simulink model "main_RI_LIEKF_GNSSOutrage"  (R2023a)
settings: Solver=FixedStepAuto  StartTime=0.0  StopTime=220  FixedStep=0.01  RelTol=1e-3
InitFcn:
  | initNavigation0612_AOA;
values from neighbouring files (symbols this model uses):
  CF_enable = 0    [initNavigation.m]
  dt = 0.01    [initNavigation.m]
  dtDelay = -0.03    [initNavigation.m]
  g0 = 9.795    [initNavigation.m]
  gam0_rad = 0/57.3    (= 0)    [initNavigation.m]
  GNSSoutragetime = 90    [initNavigation.m]
  H_sensor_type = 0    [initNavigation.m]
  KF_enable = 1    [initNavigation.m]
  P0 = diag([1*ones(3,1);0.01*ones(3,1);0.1*ones(3,1);0.001*ones(3,1);0.00001*ones(3,1)])    [initNavigation.m]
  P0_RIEKF = diag([1*ones(3,1);0.01*ones(3,1);0.1*ones(3,1);0.001*ones(3,1);0.00001*ones(3,1);      0.01*ones(3,1);[0;2;2]/57.3;[0.1;0.1;0.1]])^2    [initNavigation.m]
  pd0 = 0    [initNavigation.m]
  pe0 = 0    [initNavigation.m]
  phi0_rad = 0/57.3    (= 0)    [initNavigation.m]
  pn0 = 0    [initNavigation.m]
  psi = -178    [initNavigation.m]
  psi0_rad = 0/57.3    (= 0)    [initNavigation.m]
  state_dim = 24    [initNavigation.m]
  Time = 0:0.01:(size(traindata.AttackAngle,1) - 1)*0.01    [NNLiftCoefficientFit.m]
  vd0 = 0    [initNavigation.m]
  ve0 = 0    [initNavigation.m]
  vn0 = 0    [initNavigation.m]
undefined symbols (not defined in the file or in its folder): DiscIntNeverNeededParam, Discrete, INS_CONST, INS_EXPORT, INS_PARAM, magnitude, p, param, pInitialization, sys
libraries: simulink_extras x94, simulink x82, dspstat3 x70, sharedtransform x60, ctrlSharedLib x36, sharedTrackingLibrary x22, matrix_library x15, FMT_Model_Lib x13, deeplib x8, dspsolvers x4, vrlib x4, aerolibconvert2 x1
(part 11 of 28)

== system main_RI_LIEKF_GNSSOutrage/State estimation/LI EKF2/Error State Kalman Filter/Extended Kalman Filter1 ==
  Q : Inport
  Enable1 : Inport  Port=2
  y1 : Inport  Port=3
  R1 : Inport  Port=4
  Enable2 : Inport  Port=5
  y2 : Inport  Port=6
  R2 : Inport  Port=7
  Enable3 : Inport  Port=8
  y3 : Inport  Port=9
  R3 : Inport  Port=10
  Enable4 : Inport  Port=11
  y4 : Inport  Port=12
  R4 : Inport  Port=13
  BlockOrdering : Constant  Value=true()  OutDataTypeStr=boolean
  Correct1 : Subsystem  AncestorBlock=sharedTrackingLibrary/Extras/EKFCorrect  TreatAsAtomicUnit=on  SystemSampleTime=p.SampleTimes.MeasurementFcn(1)  mask(EKFCorrect){ProcessedMaskData=p}
      mask init: same as main_RI_LIEKF_GNSSOutrage/State estimation/0609bk/Error State Kalman Filter/Extended Kalman Filter1/Correct1
      settings: LibrarySourceBlock=sharedTrackingLibrary/Extras/EKFCorrect
  Correct2 : sharedTrackingLibrary/Extras/EKFCorrect  ProcessedMaskData=p
  Correct3 : sharedTrackingLibrary/Extras/EKFCorrect  ProcessedMaskData=p
  Correct4 : sharedTrackingLibrary/Extras/EKFCorrect  ProcessedMaskData=p
  DataStoreMemory - P : DataStoreMemory  DataStoreName=P  InitialValue=p.InitialCovariance  ShowAdditionalParam=off  OutDataTypeStr=p.DataType
  DataStoreMemory - x : DataStoreMemory  DataStoreName=x  InitialValue=p.InitialState  ShowAdditionalParam=off  OutDataTypeStr=p.DataType
  DataTypeConversion_Enable{1..4} (4 alike) : DataTypeConversion  OutDataTypeStr=boolean  SaturateOnIntegerOverflow=off  RndMeth=Floor
  DataTypeConversion_Q : DataTypeConversion  OutDataTypeStr=p.DataType  SaturateOnIntegerOverflow=off  RndMeth=Floor
  DataTypeConversion_R{1..4} (4 alike) : DataTypeConversion  OutDataTypeStr=p.DataType  SaturateOnIntegerOverflow=off  RndMeth=Floor
  DataTypeConversion_uMeas{1..4} (4 alike) : DataTypeConversion  OutDataTypeStr=p.DataType  SaturateOnIntegerOverflow=off  RndMeth=Floor
  DataTypeConversion_uState : DataTypeConversion  OutDataTypeStr=p.DataType  SaturateOnIntegerOverflow=off  RndMeth=Floor
  DataTypeConversion_y{1..4} (4 alike) : DataTypeConversion  OutDataTypeStr=p.DataType  SaturateOnIntegerOverflow=off  RndMeth=Floor
  MeasurementFcn1Inputs : Constant  Value=0  OutDataTypeStr=p.DataType  SampleTime=p.SampleTimes.MeasurementFcn(1)
  MeasurementFcn2Inputs : Constant  OutDataTypeStr=p.DataType  SampleTime=p.SampleTimes.MeasurementFcn(2)
  MeasurementFcn3Inputs : Constant  OutDataTypeStr=p.DataType  SampleTime=p.SampleTimes.MeasurementFcn(3)
  MeasurementFcn4Inputs : Constant  OutDataTypeStr=p.DataType  SampleTime=p.SampleTimes.MeasurementFcn(4)
  Output : Subsystem  TreatAsAtomicUnit=on  SystemSampleTime=p.SampleTimes.Output
  Predict : Subsystem  TreatAsAtomicUnit=on  SystemSampleTime=p.SampleTimes.StateTransitionFcn  mask(EKFPredict){ProcessedMaskData=p}
      mask init: same as main_RI_LIEKF_GNSSOutrage/State estimation/0609bk/Error State Kalman Filter/Extended Kalman Filter1/Predict
  StateTransitionFcnInputs : Constant  Value=0  OutDataTypeStr=p.DataType  SampleTime=p.SampleTimes.StateTransitionFcn
  checkMeasurementFcn1Signals : S-Function  FunctionName=ekfukfCheckSignals  Parameters=signalCheck.BlockPath, signalCheck.MeasurementFcn{1}.PortNames, signalCheck.MeasurementFcn{1}.SampleTime, signalCheck.DataType, signalCheck.MeasurementFcn{1}.PortDimensions, 1, signalCheck.MeasurementFcn{1}.HasAdditiveNoise  SFunctionDeploymentMode=off  EnableBusSupport=off
  checkMeasurementFcn2Signals : S-Function  FunctionName=ekfukfCheckSignals  Parameters=signalCheck.BlockPath, signalCheck.MeasurementFcn{2}.PortNames, signalCheck.MeasurementFcn{2}.SampleTime, signalCheck.DataType, signalCheck.MeasurementFcn{2}.PortDimensions, 1, signalCheck.MeasurementFcn{2}.HasAdditiveNoise  SFunctionDeploymentMode=off  EnableBusSupport=off
  checkMeasurementFcn3Signals : S-Function  FunctionName=ekfukfCheckSignals  Parameters=signalCheck.BlockPath, signalCheck.MeasurementFcn{3}.PortNames, signalCheck.MeasurementFcn{3}.SampleTime, signalCheck.DataType, signalCheck.MeasurementFcn{3}.PortDimensions, 1, signalCheck.MeasurementFcn{3}.HasAdditiveNoise  SFunctionDeploymentMode=off  EnableBusSupport=off
  checkMeasurementFcn4Signals : S-Function  FunctionName=ekfukfCheckSignals  Parameters=signalCheck.BlockPath, signalCheck.MeasurementFcn{4}.PortNames, signalCheck.MeasurementFcn{4}.SampleTime, signalCheck.DataType, signalCheck.MeasurementFcn{4}.PortDimensions, 1, signalCheck.MeasurementFcn{4}.HasAdditiveNoise  SFunctionDeploymentMode=off  EnableBusSupport=off
  checkStateTransitionFcnSignals : S-Function  FunctionName=ekfukfCheckSignals  Parameters=signalCheck.BlockPath, signalCheck.StateTransitionFcn.PortNames, signalCheck.StateTransitionFcn.SampleTime, signalCheck.DataType, signalCheck.StateTransitionFcn.PortDimensions, 0, signalCheck.StateTransitionFcn.HasAdditiveNoise  SFunctionDeploymentMode=off  EnableBusSupport=off
  xhat : Outport  VectorParamsAs1DForOutWhenUnconnected=off
  P : Outport  Port=2
  wires:
  Correct4/1 -> [AfterCorrect]
  Correct3/1 -> Correct4/4
  MeasurementFcn4Inputs/1 -> checkMeasurementFcn4Signals/4, DataTypeConversion_uMeas4/1
  R4/1 -> checkMeasurementFcn4Signals/3, DataTypeConversion_R4/1
  y4/1 -> checkMeasurementFcn4Signals/2, DataTypeConversion_y4/1
  Enable4/1 -> checkMeasurementFcn4Signals/1, DataTypeConversion_Enable4/1
  DataTypeConversion_uMeas4/1 -> Correct4/3
  DataTypeConversion_R4/1 -> Correct4/2
  DataTypeConversion_y4/1 -> Correct4/1
  DataTypeConversion_Enable4/1 -> Correct4/Enable
  Correct2/1 -> Correct3/4
  MeasurementFcn3Inputs/1 -> checkMeasurementFcn3Signals/4, DataTypeConversion_uMeas3/1
  R3/1 -> checkMeasurementFcn3Signals/3, DataTypeConversion_R3/1
  y3/1 -> checkMeasurementFcn3Signals/2, DataTypeConversion_y3/1
  Enable3/1 -> checkMeasurementFcn3Signals/1, DataTypeConversion_Enable3/1
  DataTypeConversion_uMeas3/1 -> Correct3/3
  DataTypeConversion_R3/1 -> Correct3/2
  DataTypeConversion_y3/1 -> Correct3/1
  DataTypeConversion_Enable3/1 -> Correct3/Enable
  Correct1/1(yBlockOrdering) -> Correct2/4
  MeasurementFcn2Inputs/1 -> checkMeasurementFcn2Signals/4, DataTypeConversion_uMeas2/1
  R2/1 -> checkMeasurementFcn2Signals/3, DataTypeConversion_R2/1
  y2/1 -> checkMeasurementFcn2Signals/2, DataTypeConversion_y2/1
  Enable2/1 -> checkMeasurementFcn2Signals/1, DataTypeConversion_Enable2/1
  DataTypeConversion_uMeas2/1 -> Correct2/3
  DataTypeConversion_R2/1 -> Correct2/2
  DataTypeConversion_y2/1 -> Correct2/1
  DataTypeConversion_Enable2/1 -> Correct2/Enable
  [AfterOutput] -> Predict/3(uBlockOrdering)
  Output/3(yBlockOrdering) -> [AfterOutput]
  [AfterCorrect] -> Output/1(uBlockOrdering)
  [FirstOperation] -> Correct1/4(uBlockOrdering)
  BlockOrdering/1 -> [FirstOperation]
  DataTypeConversion_uMeas1/1 -> Correct1/3(uMeas)
  DataTypeConversion_R1/1 -> Correct1/2(R)
  MeasurementFcn1Inputs/1 -> DataTypeConversion_uMeas1/1, checkMeasurementFcn1Signals/4
  DataTypeConversion_y1/1 -> Correct1/1(yMeas)
  DataTypeConversion_uState/1 -> Predict/2(uState)
  StateTransitionFcnInputs/1 -> DataTypeConversion_uState/1, checkStateTransitionFcnSignals/2
  Output/2(P) -> P/1
  DataTypeConversion_Enable1/1 -> Correct1/Enable
  Enable1/1 -> DataTypeConversion_Enable1/1, checkMeasurementFcn1Signals/1
  DataTypeConversion_Q/1 -> Predict/1(Q)
  Q/1 -> DataTypeConversion_Q/1, checkStateTransitionFcnSignals/1
  R1/1 -> DataTypeConversion_R1/1, checkMeasurementFcn1Signals/3
  y1/1 -> DataTypeConversion_y1/1, checkMeasurementFcn1Signals/2
  Output/1(x) -> xhat/1

== system main_RI_LIEKF_GNSSOutrage/State estimation/LI EKF2/Error State Kalman Filter/Simulink Function - GPS Measurements ==
  Rbn : Inport
  vn : Inport  Port=2
  pn : Inport  Port=3
  GPSMeasurementFcn_LIEKF : TriggerPort  TriggerType=function-call  IsSimulinkFunction=on  FunctionName=GPSMeasurementFcn_LIEKF  VariantControl=Variant
  Add : Sum
  Data Type Conversion1 : DataTypeConversion  OutDataTypeStr=single  SaturateOnIntegerOverflow=off  RndMeth=Floor
  MATLAB Function : MATLAB Function  TreatAsAtomicUnit=on
  MATLAB Function1 : MATLAB Function  Commented=on  TreatAsAtomicUnit=on
  Product : Product  Multiplication=Matrix(*)
  pn1 : InportShadow  Port=3
  vn1 : InportShadow  Port=2
  x : ArgIn  DisableCoverage=on  OutDataTypeStr=single  PortDimensions=state_dim  ArgumentName=x
  v : ArgIn  DisableCoverage=on  Port=2  OutDataTypeStr=single  PortDimensions=6  ArgumentName=v
  y : ArgOut  DisableCoverage=on  OutDataTypeStr=single  PortDimensions=6  ArgumentName=y
  wires:
  MATLAB Function/1(H) -> Data Type Conversion1/1
  Product/1 -> Add/1
  Add/1 -> y/1
  vn/1 -> MATLAB Function/1(vn)
  Rbn/1 -> MATLAB Function1/1(Rbn)
  vn1/1 -> MATLAB Function1/2(vn)
  pn1/1 -> MATLAB Function1/3(pn)
  x/1 -> Product/2
  v/1 -> Add/2
  pn/1 -> MATLAB Function/2(pn)
  Data Type Conversion1/1 -> Product/1

== system main_RI_LIEKF_GNSSOutrage/State estimation/LI EKF2/Error State Kalman Filter/Simulink Function - GPS Measurements1 ==
  vn : Inport
  pn : Inport  Port=2
  BaroMeasurementFcn_LIEKF : TriggerPort  TriggerType=function-call  IsSimulinkFunction=on  FunctionName=BaroMeasurementFcn_LIEKF  VariantControl=Variant
  Add : Sum
  Data Type Conversion1 : DataTypeConversion  OutDataTypeStr=single  SaturateOnIntegerOverflow=off  RndMeth=Floor
  MATLAB Function : MATLAB Function  TreatAsAtomicUnit=on
  Product : Product  Multiplication=Matrix(*)
  x : ArgIn  DisableCoverage=on  OutDataTypeStr=single  PortDimensions=state_dim  ArgumentName=x
  v : ArgIn  DisableCoverage=on  Port=2  OutDataTypeStr=single  ArgumentName=v
  y : ArgOut  DisableCoverage=on  OutDataTypeStr=single  ArgumentName=y
  wires:
  MATLAB Function/1(H_baro) -> Data Type Conversion1/1
  Product/1 -> Add/1
  Add/1 -> y/1
  vn/1 -> MATLAB Function/1(vn)
  x/1 -> Product/2
  v/1 -> Add/2
  pn/1 -> MATLAB Function/2(pn)
  Data Type Conversion1/1 -> Product/1

== system main_RI_LIEKF_GNSSOutrage/State estimation/LI EKF2/Error State Kalman Filter/Simulink Function - GPS Measurements2 ==
  Rbn : Inport
  Magn : Inport  Port=2
  xstate : Inport  Port=3
  MagnMeasurementFcn_LIEKF : TriggerPort  TriggerType=function-call  IsSimulinkFunction=on  FunctionName=MagnMeasurementFcn_LIEKF  VariantControl=Variant
  Add : Sum
  Data Type Conversion1 : DataTypeConversion  OutDataTypeStr=single  SaturateOnIntegerOverflow=off  RndMeth=Floor
  MATLAB Function : MATLAB Function  TreatAsAtomicUnit=on
  Product : Product  Multiplication=Matrix(*)
  Selector : Selector  InputPortWidth=state_dim  IndexOptions=Index vector (dialog)  Indices=[1 2 3]  OutputSizes=1
  x : ArgIn  DisableCoverage=on  OutDataTypeStr=single  PortDimensions=state_dim  ArgumentName=x
  v : ArgIn  DisableCoverage=on  Port=2  OutDataTypeStr=single  PortDimensions=3  ArgumentName=v
  y : ArgOut  DisableCoverage=on  OutDataTypeStr=single  PortDimensions=3  ArgumentName=y
  wires:
  MATLAB Function/1(H) -> Data Type Conversion1/1
  Product/1 -> Add/1
  Add/1 -> y/1
  Magn/1 -> MATLAB Function/2(Magn)
  x/1 -> Product/2
  v/1 -> Add/2
  Data Type Conversion1/1 -> Product/1
  Rbn/1 -> MATLAB Function/1(Rbn)
  xstate/1 -> Selector/1
  Selector/1 -> MATLAB Function/3(dtheta)

== system main_RI_LIEKF_GNSSOutrage/State estimation/LI EKF2/Error State Kalman Filter/Simulink Function - GPS Measurements3 ==
  Rbn : Inport
  vn : Inport  Port=2
  Rab : Inport  Port=3
  vel_wind_NED : Inport  Port=4
  AirspeedMeasurementFcn_LIEKF : TriggerPort  TriggerType=function-call  IsSimulinkFunction=on  FunctionName=AirspeedMeasurementFcn_LIEKF  VariantControl=Variant
  Add : Sum
  Data Type Conversion1 : DataTypeConversion  OutDataTypeStr=single  SaturateOnIntegerOverflow=off  RndMeth=Floor
  MATLAB Function : MATLAB Function  TreatAsAtomicUnit=on
  Product : Product  Multiplication=Matrix(*)
  x : ArgIn  DisableCoverage=on  OutDataTypeStr=single  PortDimensions=state_dim  ArgumentName=x
  v : ArgIn  DisableCoverage=on  Port=2  OutDataTypeStr=single  PortDimensions=3  ArgumentName=v
  y : ArgOut  DisableCoverage=on  OutDataTypeStr=single  PortDimensions=3  ArgumentName=y
  wires:
  MATLAB Function/1(H) -> Data Type Conversion1/1
  Product/1 -> Add/1
  Add/1 -> y/1
  x/1 -> Product/2
  v/1 -> Add/2
  Data Type Conversion1/1 -> Product/1
  Rbn/1 -> MATLAB Function/1(Rbn)
  vn/1 -> MATLAB Function/3(vn)
  Rab/1 -> MATLAB Function/2(Rab)
  vel_wind_NED/1 -> MATLAB Function/4(v_wind)

== system main_RI_LIEKF_GNSSOutrage/State estimation/LI EKF2/Error State Kalman Filter/Simulink Function - State Transition ==
  DCM_b_n : Inport
  wxyz : Inport  Port=2  PortDimensions=[3,1]
  axyz : Inport  Port=3  PortDimensions=[3,1]
  stateTransitionFcn_LIEKF : TriggerPort  TriggerType=function-call  IsSimulinkFunction=on  FunctionName=stateTransitionFcn_LIEKF  VariantControl=Variant
  Add : Sum
  Cal Phi : Subsystem
  Constant : Constant  Value=dt  OutDataTypeStr=single
  Data Type Conversion1 : DataTypeConversion  OutDataTypeStr=single  SaturateOnIntegerOverflow=off  RndMeth=Floor
  Data Type Conversion6 : DataTypeConversion  OutDataTypeStr=single  SaturateOnIntegerOverflow=off  RndMeth=Floor
  MATLAB Function1 : MATLAB Function  TreatAsAtomicUnit=on
  Product1 : Product  Multiplication=Matrix(*)
  Product2 : Product  Multiplication=Matrix(*)
  x : ArgIn  DisableCoverage=on  OutDataTypeStr=single  PortDimensions=state_dim  ArgumentName=x
  w : ArgIn  Port=2  OutDataTypeStr=single  PortDimensions=cov_dim  ArgumentName=w
  xNext : ArgOut  DisableCoverage=on  OutDataTypeStr=single  PortDimensions=state_dim  ArgumentName=xNext
  wires:
  x/1 -> Product2/2
  Product2/1 -> Data Type Conversion6/1
  MATLAB Function1/1(G) -> Product1/1
  w/1 -> Product1/2
  Product1/1 -> Data Type Conversion1/1
  Add/1 -> xNext/1
  [DCM_b_n] -> MATLAB Function1/1(Rbn)
  Constant/1 -> MATLAB Function1/2(dt)
  DCM_b_n/1 -> [DCM_b_n]
  Cal Phi/1(Phi) -> Product2/1
  Data Type Conversion6/1 -> Add/2
  [DCM_b_n] -> Cal Phi/1(Rbn)
  wxyz/1 -> Cal Phi/2(wxyz)
  axyz/1 -> Cal Phi/3(axyz)
  Data Type Conversion1/1 -> Add/1

== system main_RI_LIEKF_GNSSOutrage/State estimation/LI EKF2/Error State Kalman Filter/Simulink Function - State Transition1 ==
  DCM_b_n : Inport
  wxyz : Inport  Port=2  PortDimensions=[3,1]
  axyz : Inport  Port=3  PortDimensions=[3,1]
  stateFcn_LIEKFJacobian : TriggerPort  TriggerType=function-call  IsSimulinkFunction=on  FunctionName=stateFcn_LIEKFJacobian  VariantControl=Variant
  Cal Phi : Subsystem
  Constant : Constant  Value=dt  OutDataTypeStr=single
  Data Type Conversion1 : DataTypeConversion  OutDataTypeStr=single  SaturateOnIntegerOverflow=off  RndMeth=Floor
  Data Type Conversion6 : DataTypeConversion  OutDataTypeStr=single  SaturateOnIntegerOverflow=off  RndMeth=Floor
  MATLAB Function1 : MATLAB Function  TreatAsAtomicUnit=on
  Terminator : Terminator
  Terminator1 : Terminator
  x : ArgIn  DisableCoverage=on  OutDataTypeStr=single  PortDimensions=state_dim  ArgumentName=x
  w : ArgIn  Port=2  OutDataTypeStr=single  PortDimensions=cov_dim  ArgumentName=w
  A : ArgOut  DisableCoverage=on  OutDataTypeStr=single  PortDimensions=[state_dim,state_dim]  ArgumentName=A
  G : ArgOut  Port=2  OutDataTypeStr=single  PortDimensions=[24,21]  ArgumentName=G
  wires:
  axyz/1 -> Cal Phi/3(a)
  wxyz/1 -> Cal Phi/2(w)
  [DCM_b_n] -> Cal Phi/1(Rbn)
  DCM_b_n/1 -> [DCM_b_n]
  Constant/1 -> MATLAB Function1/2(dt)
  [DCM_b_n] -> MATLAB Function1/1(Rbn)
  w/1 -> Terminator/1
  x/1 -> Terminator1/1
  MATLAB Function1/1(G) -> Data Type Conversion6/1
  Cal Phi/1(Phi) -> Data Type Conversion1/1
  Data Type Conversion6/1 -> G/1
  Data Type Conversion1/1 -> A/1

== system main_RI_LIEKF_GNSSOutrage/State estimation/LI EKF2/Error State Kalman Filter/Subsystem ==
  data : Inport
  Detect Change : simulink/Logic and Bit Operations/Detect Change  vinit=0  InputProcessing=Columns as channels (frame based)  OutDataTypeStr=boolean
  Selector : Selector  InputPortWidth=3  IndexOptions=Index vector (dialog)  Indices=[3]  OutputSizes=1
  Zero-Order Hold : ZeroOrderHold  SampleTime=0.2
  Zero-Order Hold1 : ZeroOrderHold  SampleTime=0.01
  flag : Outport
  wires:
  Zero-Order Hold1/1 -> Detect Change/1
  Detect Change/1 -> flag/1
  Selector/1 -> Zero-Order Hold1/1
  data/1 -> Zero-Order Hold/1
  Zero-Order Hold/1 -> Selector/1

== system main_RI_LIEKF_GNSSOutrage/State estimation/LI EKF2/Error State Kalman Filter/Subsystem1 ==
  Cbn : Inport
  v_I : Inport  Port=2
  v_G : Inport  Port=3
  p_I : Inport  Port=4
  p_G : Inport  Port=5
  Add1 : Sum  Inputs=+-
  Add2 : Sum  Inputs=+-
  Data Type Conversion : DataTypeConversion  OutDataTypeStr=single  SaturateOnIntegerOverflow=off  RndMeth=Floor
  Data Type Conversion2 : DataTypeConversion  OutDataTypeStr=single  SaturateOnIntegerOverflow=off  RndMeth=Floor
  Gain1 : Gain  Gain=-1
  Mux2 : Mux  Inputs=2
  Product : Product  Multiplication=Matrix(*)
  Product1 : Product  Multiplication=Matrix(*)
  Transpose : Math  Operator=transpose
  dv/dp : Outport
  wires:
  Gain1/1 -> dv/dp/1
  Mux2/1 -> Gain1/1
  Product1/1 -> Data Type Conversion/1
  Product/1 -> Data Type Conversion2/1
  Transpose/1 -> Product1/1, Product/1
  Cbn/1 -> Transpose/1
  Data Type Conversion2/1 -> Mux2/1
  v_G/1 -> Add2/2
  Data Type Conversion/1 -> Mux2/2
  p_I/1 -> Add1/1
  Add1/1 -> Product1/2
  Add2/1 -> Product/2
  v_I/1 -> Add2/1
  p_G/1 -> Add1/2

== system main_RI_LIEKF_GNSSOutrage/State estimation/LI EKF2/Error State Kalman Filter/Subsystem2 ==
  p_INS : Inport
  H_baro : Inport  Port=2
  Add : Sum
  dpZ : Outport
  wires:
  p_INS/1 -> Add/1
  H_baro/1 -> Add/2
  Add/1 -> dpZ/1

== system main_RI_LIEKF_GNSSOutrage/State estimation/LI EKF2/Error State Kalman Filter/Subsystem3 ==
  data : Inport
  Detect Change : simulink/Logic and Bit Operations/Detect Change  vinit=0  InputProcessing=Columns as channels (frame based)  OutDataTypeStr=boolean
  From Workspace1 : FromWorkspace  Commented=on  VariableName=[All.t',All.vn]
  From Workspace7 : FromWorkspace  VariableName=[All.t',All.lat]
  Selector : Selector  InputPortWidth=3  IndexOptions=Index vector (dialog)  Indices=[3]  OutputSizes=1
  flag : Outport
  wires:
  Detect Change/1 -> flag/1
  data/1 -> Selector/1
  From Workspace7/1 -> Detect Change/1  "lat"

== system main_RI_LIEKF_GNSSOutrage/State estimation/LI EKF2/Error State Kalman Filter/bak ==
  From1 : From  Commented=on  GotoTag=wxyz
  From11 : From  Commented=on  GotoTag=p_INS
  From14 : From  Commented=on  GotoTag=DCM_b_n
  From2 : From  Commented=on  GotoTag=fbxyz
  From3 : From  Commented=on  GotoTag=ZUPTenable
  From4 : From  Commented=on  GotoTag=v_INS
  From5 : From  Commented=on  GotoTag=fex
  From6 : From  Commented=on  GotoTag=DCM_b_n
  From9 : From  Commented=on  GotoTag=DCM_b_n
  Goto6 : Goto  Commented=on  GotoTag=ZUPTenable
  MATLAB Function1 : MATLAB Function  Commented=on  TreatAsAtomicUnit=on
  Memory1 : Memory  Commented=on
  RIEKF : MATLAB Function  Commented=on  TreatAsAtomicUnit=on
  Rate Transition2 : RateTransition  Commented=on  OutPortSampleTime=dt
  Scope10 : Scope  Commented=on  NumInputPorts=2
  Simulink Function - GPS Measurements1 : Subsystem  Commented=on  TreatAsAtomicUnit=on
  Simulink Function - GPS Measurements2 : Subsystem  Commented=on  TreatAsAtomicUnit=on
  Simulink Function - State Transition Jacobian : Subsystem  Commented=on  TreatAsAtomicUnit=on
  Unscented Kalman Filter1 : sharedTrackingLibrary/Unscented Kalman Filter  Commented=on  StateTransitionFcn=stateTransitionFcn_Dyn  HasAdditiveProcessNoise=Nonadditive  ProcessNoise=1  HasTimeVaryingProcessNoise=on  HasStateTransitionFcnExtraArgument=0  InitialState=zeros(18,1)  InitialStateCovariance=diag([1*ones(3,1);0.1*ones(3,1);0.001*ones(3,1);0.001*ones(6,1);0.1*ones(3,1)]);  Alpha=1e-2  Beta=2  Kappa=0  MeasurementFcn1=GPSMeasurementFcn_Dyn  HasMeasurementEnablePort1=on  HasAdditiveMeasurementNoise1=Nonadditive  MeasurementNoise1=1  HasTimeVaryingMeasurementNoise1=on  HasMeasurementFcnExtraArgument1=0  HasMeasurementWrapping1=off  MeasurementFcn2=DynamicMeasurementFcn_Dyn  HasMeasurementEnablePort2=on  HasAdditiveMeasurementNoise2=Nonadditive  MeasurementNoise2=1  HasTimeVaryingMeasurementNoise2=on  HasMeasurementFcnExtraArgument2=0  HasMeasurementWrapping2=off  MeasurementFcn3=myMeasurementFcn  HasMeasurementEnablePort3=off  HasAdditiveMeasurementNoise3=Additive  MeasurementNoise3=1  HasTimeVaryingMeasurementNoise3=off  HasMeasurementFcnExtraArgument3=0  HasMeasurementWrapping3=off  MeasurementFcn4=myMeasurementFcn  HasMeasurementEnablePort4=off  HasAdditiveMeasurementNoise4=Additive  MeasurementNoise4=1  HasTimeVaryingMeasurementNoise4=off  HasMeasurementFcnExtraArgument4=0  HasMeasurementWrapping4=off  MeasurementFcn5=myMeasurementFcn  HasMeasurementEnablePort5=off  HasAdditiveMeasurementNoise5=Additive  MeasurementNoise5=1  HasTimeVaryingMeasurementNoise5=off  HasMeasurementFcnExtraArgument5=0  HasMeasurementWrapping5=off  EnableMultirate=off  StateTransitionFcnSampleTime=1  MeasurementFcn1SampleTime=1  MeasurementFcn2SampleTime=1  MeasurementFcn3SampleTime=1  MeasurementFcn4SampleTime=1  MeasurementFcn5SampleTime=1  UseCurrentEstimator=on  OutputStateCovariance=on  DataType=single  SampleTime=0.01  NumberOfMeasurements=2
  Out1 : Outport
  wires:
  Memory1/1 -> MATLAB Function1/4(fex)
  Rate Transition2/1 -> Out1/1
  From1/1 -> MATLAB Function1/2(wxyz)
  MATLAB Function1/1(ZeroVelDetectFlag) -> Scope10/1, Goto6/1
  From5/1 -> Memory1/1
  From2/1 -> MATLAB Function1/3(fbxyz)
  From6/1 -> MATLAB Function1/1(Cbn)
  MATLAB Function1/2(ZeroVelDetectFlagold) -> Scope10/2
  From3/1 -> Rate Transition2/1
  From11/1 -> Simulink Function - State Transition Jacobian/3(pn)
  From9/1 -> Simulink Function - State Transition Jacobian/1(DCM_b_n)
  From4/1 -> Simulink Function - State Transition Jacobian/2(vn)
  From14/1 -> Simulink Function - GPS Measurements1/1(DCM_b_n)

== system main_RI_LIEKF_GNSSOutrage/State estimation/LI EKF2/INS propogation/AOA//SA//Vwind update ==
  note: The total Velocity > 10m/s
  INSstate_v : Inport
  vel_NED : Inport  Port=2
  Cbn : Inport  Port=3
  dtheta_a : Inport  Port=4
  TAS : Inport  Port=5
  dv_wind : Inport  Port=6
  gyro_raw : Inport  Port=7
  accl_raw : Inport  Port=8
  elevator_aileron_rudder_deg : Inport  Port=9
  Constant : Constant  Value=eye(3)
  Memory : Memory
  Subsystem : Subsystem
  Subsystem1 : Subsystem
  Subsystem2 : Subsystem
  Switch : Switch  Threshold=1  SaturateOnIntegerOverflow=off  InputSameDT=off
  INSstate_Rab : Outport
  vel_wind : Outport  Port=2
  wires:
  Constant/1 -> Switch/3
  dtheta_a/1 -> Subsystem/5(dtheta_a)
  Subsystem/1(INSstate_Rab) -> Switch/1, Subsystem2/2(INSstate_Rab)  "INSstate_Rab"
  INSstate_v/1 -> Subsystem2/3(INSstate_v), Subsystem/2(vel_NED)
  vel_NED/1 -> Subsystem1/1(vel_NED)
  Subsystem1/1(AOA_Estimation_flag) -> Switch/2, Subsystem2/Enable, Subsystem/Enable
  Cbn/1 -> Subsystem2/1(Rbn), Subsystem/1(Cbn)
  Subsystem2/1(v_wind_out) -> Memory/1, vel_wind/1  "vel_wind"
  Switch/1 -> INSstate_Rab/1  "INSstate_Rab"
  TAS/1 -> Subsystem/8(TAS), Subsystem2/4(TAS)
  dv_wind/1 -> Subsystem2/5(dv_wind)
  Memory/1 -> Subsystem/3(vel_wind_NED)
  elevator_aileron_rudder_deg/1 -> Subsystem/6(elevator_aileron_rudder_deg)
  gyro_raw/1 -> Subsystem/4(gyro_raw)
  accl_raw/1 -> Subsystem/7(accl_raw)

== system main_RI_LIEKF_GNSSOutrage/State estimation/LI EKF2/INS propogation/Init_PVQ ==
  QGC_sensor_reinit : Inport
  accl_B_m/s2_LPF : Inport  Port=2
  Magn_B_guess_LPF : Inport  Port=3
  pos_NED : Inport  Port=4
  vel_NED : Inport  Port=5
  Add : Sum
  Add1 : Sum
  Constant : Constant  Value=[1 0 0 0]  OutDataTypeStr=single
  Constant1 : Constant  OutDataTypeStr=uint8
  Constant2 : Constant  Value=[0;0;0]  OutDataTypeStr=single
  Constant3 : Constant  Value=[0;0;0]  OutDataTypeStr=single
  Constant4 : Constant  Value=[vn0;ve0;vd0]  OutDataTypeStr=single
  Constant5 : Constant  Value=[pn0;pe0;pd0]  OutDataTypeStr=single
  Detect Increase : simulink/Logic and Bit Operations/Detect Increase  vinit=0.0  OutDataTypeStr=boolean
  Horizontal_attitude1 : Subsystem  TreatAsAtomicUnit=on
  Horizontal_attitude2 : Subsystem  Commented=on  TreatAsAtomicUnit=on
  Memory : Memory
  Scope : Scope  NumInputPorts=2
  Scope1 : Scope
  Subsystem : Subsystem
  Subsystem1 : Subsystem
  Switch{,1..3} (4 alike) : Switch  Criteria=u2 > Threshold  SaturateOnIntegerOverflow=off  InputSameDT=off
  quat_0 : Outport
  v0 : Outport  Port=2
  p0 : Outport  Port=3
  wires:
  Add/1 -> Switch2/1
  Add1/1 -> Switch3/1
  Switch3/1 -> p0/1
  Switch2/1 -> v0/1
  Constant3/1 -> Switch3/3
  Constant2/1 -> Switch2/3
  Detect Increase/1 -> Scope/2, Switch1/2, Horizontal_attitude1/Enable
  Magn_B_guess_LPF/1 -> Subsystem1/1(data)
  QGC_sensor_reinit/1 -> Scope/1, Detect Increase/1
  accl_B_m/s2_LPF/1 -> Subsystem/1(data)
  Switch1/1 -> Scope1/1, Switch/2, Switch3/2, Switch2/2, Memory/1
  Constant1/1 -> Switch1/1
  Horizontal_attitude1/1(quat_0) -> Switch/1
  Constant/1 -> Switch/3
  Memory/1 -> Switch1/3
  Subsystem/1(mean_data) -> Horizontal_attitude1/1(accl_mean_B_m/s_LPF)
  Subsystem1/1(mean_data) -> Horizontal_attitude1/2(Magn_mean_B_guess_LPF)
  Switch/1 -> quat_0/1
  vel_NED/1 -> Add/1
  Constant4/1 -> Add/2
  Constant5/1 -> Add1/2
  pos_NED/1 -> Add1/1

== system main_RI_LIEKF_GNSSOutrage/State estimation/LI EKF2/INS propogation/accl bias compensation ==
  QGC_init : Inport
  raw <accl_B_m/s2_LPF> : Inport  Port=2
  dda : Inport  Port=3
  Add2 : Sum
  Data Type Conversion6 : DataTypeConversion  OutDataTypeStr=single  SaturateOnIntegerOverflow=off  RndMeth=Floor
  Scope : Scope
  error compensation1 : Subsystem
  fb : Outport  PortDimensions=3
  da : Outport  Port=2  PortDimensions=3
  wires:
  dda/1 -> error compensation1/1(dda)
  raw <accl_B_m/s2_LPF>/1 -> Add2/1
  Data Type Conversion6/1 -> fb/1
  Add2/1 -> Data Type Conversion6/1
  error compensation1/1(da) -> Add2/2, da/1, Scope/1
  QGC_init/1 -> error compensation1/2(QGC_init)

== system main_RI_LIEKF_GNSSOutrage/State estimation/LI EKF2/INS propogation/accl bias compensation1 ==
  QGC_init : Inport
  raw <accl_B_m/s2_LPF> : Inport  Port=2
  dda : Inport  Port=3
  Add2 : Sum
  Bus Selector : BusSelector  OutputSignals=mag_norm_B
  Data Type Conversion6 : DataTypeConversion  OutDataTypeStr=single  SaturateOnIntegerOverflow=off  RndMeth=Floor
  error compensation1 : Subsystem
  mgan : Outport  PortDimensions=3
  dm : Outport  Port=2  PortDimensions=3
  wires:
  raw <accl_B_m/s2_LPF>/1 -> Bus Selector/1
  QGC_init/1 -> error compensation1/2(QGC_init)
  error compensation1/1(da) -> dm/1, Add2/2
  Add2/1 -> Data Type Conversion6/1
  Data Type Conversion6/1 -> mgan/1
  Bus Selector/1 -> Add2/1  "<mag_norm_B>"
  dda/1 -> error compensation1/1(dda)

== system main_RI_LIEKF_GNSSOutrage/State estimation/LI EKF2/INS propogation/accl bias compensation2 ==
  QGC_init : Inport
  dda : Inport  Port=2
  Enable : EnablePort
  Data Type Conversion6 : DataTypeConversion  OutDataTypeStr=single  SaturateOnIntegerOverflow=off  RndMeth=Floor
  error compensation1 : Subsystem
  v : Outport
  wires:
  dda/1 -> error compensation1/1(dda)
  Data Type Conversion6/1 -> v/1
  error compensation1/1(da) -> Data Type Conversion6/1
  QGC_init/1 -> error compensation1/2(QGC_init)

== system main_RI_LIEKF_GNSSOutrage/State estimation/LI EKF2/INS propogation/att update ==
  dtheta : Inport
  gyro : Inport  Port=2
  quat_0 : Inport  Port=3  PortDimensions=4
  init_flag : Inport  Port=4
  Bus Creator1 : BusCreator  Inputs=1
  Constant : Constant  Value=dt
  Delay1 : Delay  DelayLength=1  InitialConditionSource=Input port  InitialCondition=0  ExternalReset=Level hold
      settings: InputPortMap=u0,r5,p4
  Detect Increase : simulink/Logic and Bit Operations/Detect Increase  vinit=0.0  OutDataTypeStr=boolean
  Gain1 : Gain  Gain=[1;1;-1]
  MATLAB Function : MATLAB Function  TreatAsAtomicUnit=on
  MATLAB Function2 : MATLAB Function  TreatAsAtomicUnit=on
  Quaternions to Direction Cosine Matrix : sharedtransform/Quaternions to  Direction Cosine Matrix  aMode=aMode
      settings: LibrarySourceBlock=|
      | aerolibtransform2/Quaternions to
      | Direction Cosine Matrix
  Saturation1 : Saturate  Commented=on  UpperLimit=[1;1;1]*0.01  LowerLimit=-[1;1;1]*0.01
  Scope : Scope
  Transpose : Math  Operator=transpose
  att_update1 : Outport
  wires:
  Gain1/1 -> Scope/1, MATLAB Function2/1(delta)
  dtheta/1 -> Gain1/1
  init_flag/1 -> Detect Increase/1
  quat_0/1 -> Quaternions to Direction Cosine Matrix/1
  gyro/1 -> MATLAB Function/2(w)  "w"
  Constant/1 -> MATLAB Function/3(dt)
  Quaternions to Direction Cosine Matrix/1 -> Transpose/1
  Transpose/1 -> Delay1/3
  Delay1/1 -> MATLAB Function/1(Rbn_k_1)
  Detect Increase/1 -> Delay1/2
  Bus Creator1/1 -> att_update1/1
  MATLAB Function/1(Rbn) -> MATLAB Function2/2(Rbn)  "DCM_b_n"
  MATLAB Function2/1(Rbn_correct) -> Bus Creator1/1, Delay1/1  "DCM_b_n"

== system main_RI_LIEKF_GNSSOutrage/State estimation/LI EKF2/INS propogation/gyro bias compensation ==
  raw <gyro_B_rad/s_LPF> : Inport
  ddg : Inport  Port=2
  Measuemrnt Enable Flag : Inport  Port=3
  QGC_init : Inport  Port=4
  Add1 : Sum
  Data Type Conversion4 : DataTypeConversion  OutDataTypeStr=single  SaturateOnIntegerOverflow=off  RndMeth=Floor
  Scope1 : Scope
  error compensation : Subsystem
      settings: PortSchema="{\"entries\":[{\"content\":{\"sides\":[{\"content\":{\"connectorIds\":[\"In1\",\"In2\"]},\"type\":\"ConnectorPlacement.EquallySpacedRectSide\",\"uuid\":\"380e61a1-8124-48da-8c16-e78a4b6c30a9\"},{\"content\":{\"connectorIds\":[\"Out1\"],\"side\":\"RIGHT\"},\"type\":\"ConnectorPlacement.EquallySpacedRectSide\",\"uuid\":\"dacfd24e-67c3-4852-b5f7-795187362148\"},{\"content\":{\"side\":\"TOP\"},\"type\":\"ConnectorPlacement.EquallySpacedRectSide\",\"uuid\":\"56579dc4-3963-4476-a5d7-e0c30cfcd11c\"},{\"content\":{\"connectorIds\":[\"In3\"],\"side\":\"BOTTOM\"},\"type\":\"ConnectorPlacement.EquallySpacedRectSide\",\"uuid\":\"fc24e139-e918-40f2-99cc-0ca16c0a4a58\"}]},\"type\":\"ConnectorPlacement.EquallySpacedConnector\",\"uuid\":\"3ce5c04a-f8d2-476b-8ef1-0541292dfd95\"}],\"packageUris\":[\"http://schema.mathworks.com/mf0/Connector/R2020b\"],\"version\":\"1.0\"}"
  wb : Outport  PortDimensions=3
  dg : Outport  Port=2  PortDimensions=3
  wires:
  Data Type Conversion4/1 -> wb/1
  raw <gyro_B_rad/s_LPF>/1 -> Add1/1
  error compensation/1(dg) -> Add1/2, Scope1/1, dg/1
  Measuemrnt Enable Flag/1 -> error compensation/2(Enable)
  Add1/1 -> Data Type Conversion4/1
  QGC_init/1 -> error compensation/3(QGC_init)
  ddg/1 -> error compensation/1(ddg)

== system main_RI_LIEKF_GNSSOutrage/State estimation/LI EKF2/INS propogation/vel//pos update ==
  dtheta : Inport
  <DCM_b_n> : Inport  Port=2
  Ab : Inport  Port=3
  v0 : Inport  Port=4
  p0 : Inport  Port=5
  QGC_init : Inport  Port=6
  dp : Inport  Port=7
  dv : Inport  Port=8
  Add : Sum
  Add1 : Sum
  Add2 : Sum
  Constant : Constant  Value=[-0.45;0;0]  OutDataTypeStr=single
  Constant1 : Constant  Value=dtDelay  OutDataTypeStr=single
  Constant2 : Constant  Value=dtDelay  OutDataTypeStr=single
  Kinematic Equation : Subsystem
  Product : Product  Multiplication=Matrix(*)
  Product1 : Product
  Product2 : Product
  QGC_init1 : InportShadow  Port=6
  pos update : Subsystem
  vel update : Subsystem
  p_k : Outport  PortDimensions=3
  V : Outport  Port=2  PortDimensions=3
  pL_k : Outport  Port=3  PortDimensions=3
  VL : Outport  Port=4  PortDimensions=3
  wires:
  Add2/1 -> pL_k/1
  Product2/1 -> Add2/1
  Constant2/1 -> Product2/1
  Add1/1 -> VL/1, Product2/2
  Constant1/1 -> Product1/1
  Product1/1 -> Add1/1
  Add/1 -> Add2/2
  <DCM_b_n>/1 -> pos update/6(<DCM_b_n>), vel update/6(Cbn), Kinematic Equation/1(Cbn), Product/1
  Constant/1 -> Product/2
  Product/1 -> Add/2
  pos update/1(p_k) -> p_k/1, Add/1
  QGC_init1/1 -> pos update/4(QGC_init)
  p0/1 -> pos update/5(p0)
  dp/1 -> pos update/3(dp)
  v0/1 -> vel update/5(v0)
  dv/1 -> vel update/4(KFState_dv)
  Kinematic Equation/1(An) -> vel update/3(An), Product1/2
  QGC_init/1 -> vel update/2(QGC_init)
  Ab/1 -> Kinematic Equation/2(Ab)
  vel update/1(vel_k) -> V/1, pos update/2(vel_k), Add1/2
  dtheta/1 -> vel update/1(dtheta), pos update/1(dtheta)

== system main_RI_LIEKF_GNSSOutrage/State estimation/RI EKF_AOA_LSTM/Error State Kalman Filter/Cal Q1 ==
  Constant : Constant  Value=dt  OutDataTypeStr=double
  MATLAB Function1 : MATLAB Function  TreatAsAtomicUnit=on
  Qd : Outport
  wires:
  Constant/1 -> MATLAB Function1/1(dt)
  MATLAB Function1/1(Q) -> Qd/1

== system main_RI_LIEKF_GNSSOutrage/State estimation/RI EKF_AOA_LSTM/Error State Kalman Filter/Extended Kalman Filter1 ==
  Q : Inport
  Enable1 : Inport  Port=2
  y1 : Inport  Port=3
  R1 : Inport  Port=4
  Enable2 : Inport  Port=5
  y2 : Inport  Port=6
  R2 : Inport  Port=7
  Enable3 : Inport  Port=8
  y3 : Inport  Port=9
  R3 : Inport  Port=10
  Enable4 : Inport  Port=11
  y4 : Inport  Port=12
  R4 : Inport  Port=13
  BlockOrdering : Constant  Value=true()  OutDataTypeStr=boolean
  Correct1 : Subsystem  AncestorBlock=sharedTrackingLibrary/Extras/EKFCorrect  TreatAsAtomicUnit=on  SystemSampleTime=p.SampleTimes.MeasurementFcn(1)  mask(EKFCorrect){ProcessedMaskData=p}
      mask init: same as main_RI_LIEKF_GNSSOutrage/State estimation/0609bk/Error State Kalman Filter/Extended Kalman Filter1/Correct1
      settings: LibrarySourceBlock=sharedTrackingLibrary/Extras/EKFCorrect
  Correct2 : sharedTrackingLibrary/Extras/EKFCorrect  ProcessedMaskData=p
  Correct3 : sharedTrackingLibrary/Extras/EKFCorrect  ProcessedMaskData=p
  Correct4 : sharedTrackingLibrary/Extras/EKFCorrect  ProcessedMaskData=p
  DataStoreMemory - P : DataStoreMemory  DataStoreName=P  InitialValue=p.InitialCovariance  ShowAdditionalParam=off  OutDataTypeStr=p.DataType
  DataStoreMemory - x : DataStoreMemory  DataStoreName=x  InitialValue=p.InitialState  ShowAdditionalParam=off  OutDataTypeStr=p.DataType
  DataTypeConversion_Enable{1..4} (4 alike) : DataTypeConversion  OutDataTypeStr=boolean  SaturateOnIntegerOverflow=off  RndMeth=Floor
  DataTypeConversion_Q : DataTypeConversion  OutDataTypeStr=p.DataType  SaturateOnIntegerOverflow=off  RndMeth=Floor
  DataTypeConversion_R{1..4} (4 alike) : DataTypeConversion  OutDataTypeStr=p.DataType  SaturateOnIntegerOverflow=off  RndMeth=Floor
  DataTypeConversion_uMeas{1..4} (4 alike) : DataTypeConversion  OutDataTypeStr=p.DataType  SaturateOnIntegerOverflow=off  RndMeth=Floor
  DataTypeConversion_uState : DataTypeConversion  OutDataTypeStr=p.DataType  SaturateOnIntegerOverflow=off  RndMeth=Floor
  DataTypeConversion_y{1..4} (4 alike) : DataTypeConversion  OutDataTypeStr=p.DataType  SaturateOnIntegerOverflow=off  RndMeth=Floor
  MeasurementFcn1Inputs : Constant  Value=0  OutDataTypeStr=p.DataType  SampleTime=p.SampleTimes.MeasurementFcn(1)
  MeasurementFcn2Inputs : Constant  OutDataTypeStr=p.DataType  SampleTime=p.SampleTimes.MeasurementFcn(2)
  MeasurementFcn3Inputs : Constant  OutDataTypeStr=p.DataType  SampleTime=p.SampleTimes.MeasurementFcn(3)
  MeasurementFcn4Inputs : Constant  OutDataTypeStr=p.DataType  SampleTime=p.SampleTimes.MeasurementFcn(4)
  Output : Subsystem  TreatAsAtomicUnit=on  SystemSampleTime=p.SampleTimes.Output
  Predict : Subsystem  TreatAsAtomicUnit=on  SystemSampleTime=p.SampleTimes.StateTransitionFcn  mask(EKFPredict){ProcessedMaskData=p}
      mask init: same as main_RI_LIEKF_GNSSOutrage/State estimation/0609bk/Error State Kalman Filter/Extended Kalman Filter1/Predict
  StateTransitionFcnInputs : Constant  Value=0  OutDataTypeStr=p.DataType  SampleTime=p.SampleTimes.StateTransitionFcn
  checkMeasurementFcn1Signals : S-Function  FunctionName=ekfukfCheckSignals  Parameters=signalCheck.BlockPath, signalCheck.MeasurementFcn{1}.PortNames, signalCheck.MeasurementFcn{1}.SampleTime, signalCheck.DataType, signalCheck.MeasurementFcn{1}.PortDimensions, 1, signalCheck.MeasurementFcn{1}.HasAdditiveNoise  SFunctionDeploymentMode=off  EnableBusSupport=off
  checkMeasurementFcn2Signals : S-Function  FunctionName=ekfukfCheckSignals  Parameters=signalCheck.BlockPath, signalCheck.MeasurementFcn{2}.PortNames, signalCheck.MeasurementFcn{2}.SampleTime, signalCheck.DataType, signalCheck.MeasurementFcn{2}.PortDimensions, 1, signalCheck.MeasurementFcn{2}.HasAdditiveNoise  SFunctionDeploymentMode=off  EnableBusSupport=off
  checkMeasurementFcn3Signals : S-Function  FunctionName=ekfukfCheckSignals  Parameters=signalCheck.BlockPath, signalCheck.MeasurementFcn{3}.PortNames, signalCheck.MeasurementFcn{3}.SampleTime, signalCheck.DataType, signalCheck.MeasurementFcn{3}.PortDimensions, 1, signalCheck.MeasurementFcn{3}.HasAdditiveNoise  SFunctionDeploymentMode=off  EnableBusSupport=off
  checkMeasurementFcn4Signals : S-Function  FunctionName=ekfukfCheckSignals  Parameters=signalCheck.BlockPath, signalCheck.MeasurementFcn{4}.PortNames, signalCheck.MeasurementFcn{4}.SampleTime, signalCheck.DataType, signalCheck.MeasurementFcn{4}.PortDimensions, 1, signalCheck.MeasurementFcn{4}.HasAdditiveNoise  SFunctionDeploymentMode=off  EnableBusSupport=off
  checkStateTransitionFcnSignals : S-Function  FunctionName=ekfukfCheckSignals  Parameters=signalCheck.BlockPath, signalCheck.StateTransitionFcn.PortNames, signalCheck.StateTransitionFcn.SampleTime, signalCheck.DataType, signalCheck.StateTransitionFcn.PortDimensions, 0, signalCheck.StateTransitionFcn.HasAdditiveNoise  SFunctionDeploymentMode=off  EnableBusSupport=off
  xhat : Outport  VectorParamsAs1DForOutWhenUnconnected=off
  P : Outport  Port=2
  wires:
  [AfterOutput] -> Predict/3(uBlockOrdering)
  Output/3(yBlockOrdering) -> [AfterOutput]
  [AfterCorrect] -> Output/1(uBlockOrdering)
  [FirstOperation] -> Correct1/4(uBlockOrdering)
  BlockOrdering/1 -> [FirstOperation]
  DataTypeConversion_uMeas1/1 -> Correct1/3(uMeas)
  DataTypeConversion_R1/1 -> Correct1/2(R)
  MeasurementFcn1Inputs/1 -> DataTypeConversion_uMeas1/1, checkMeasurementFcn1Signals/4
  DataTypeConversion_y1/1 -> Correct1/1(yMeas)
  DataTypeConversion_uState/1 -> Predict/2(uState)
  StateTransitionFcnInputs/1 -> DataTypeConversion_uState/1, checkStateTransitionFcnSignals/2
  Output/2(P) -> P/1
  DataTypeConversion_Enable1/1 -> Correct1/Enable
  Enable1/1 -> DataTypeConversion_Enable1/1, checkMeasurementFcn1Signals/1
  DataTypeConversion_Q/1 -> Predict/1(Q)
  Q/1 -> DataTypeConversion_Q/1, checkStateTransitionFcnSignals/1
  R1/1 -> DataTypeConversion_R1/1, checkMeasurementFcn1Signals/3
  y1/1 -> DataTypeConversion_y1/1, checkMeasurementFcn1Signals/2
  Output/1(x) -> xhat/1
  DataTypeConversion_Enable2/1 -> Correct2/Enable
  DataTypeConversion_y2/1 -> Correct2/1
  DataTypeConversion_R2/1 -> Correct2/2
  DataTypeConversion_uMeas2/1 -> Correct2/3
  Enable2/1 -> DataTypeConversion_Enable2/1, checkMeasurementFcn2Signals/1
  y2/1 -> DataTypeConversion_y2/1, checkMeasurementFcn2Signals/2
  R2/1 -> DataTypeConversion_R2/1, checkMeasurementFcn2Signals/3
  MeasurementFcn2Inputs/1 -> DataTypeConversion_uMeas2/1, checkMeasurementFcn2Signals/4
  Correct1/1(yBlockOrdering) -> Correct2/4
  DataTypeConversion_Enable3/1 -> Correct3/Enable
  DataTypeConversion_y3/1 -> Correct3/1
  DataTypeConversion_R3/1 -> Correct3/2
  DataTypeConversion_uMeas3/1 -> Correct3/3
  Enable3/1 -> DataTypeConversion_Enable3/1, checkMeasurementFcn3Signals/1
  y3/1 -> DataTypeConversion_y3/1, checkMeasurementFcn3Signals/2
  R3/1 -> DataTypeConversion_R3/1, checkMeasurementFcn3Signals/3
  MeasurementFcn3Inputs/1 -> DataTypeConversion_uMeas3/1, checkMeasurementFcn3Signals/4
  Correct2/1 -> Correct3/4
  DataTypeConversion_Enable4/1 -> Correct4/Enable
  DataTypeConversion_y4/1 -> Correct4/1
  DataTypeConversion_R4/1 -> Correct4/2
  DataTypeConversion_uMeas4/1 -> Correct4/3
  Enable4/1 -> DataTypeConversion_Enable4/1, checkMeasurementFcn4Signals/1
  y4/1 -> DataTypeConversion_y4/1, checkMeasurementFcn4Signals/2
  R4/1 -> DataTypeConversion_R4/1, checkMeasurementFcn4Signals/3
  MeasurementFcn4Inputs/1 -> DataTypeConversion_uMeas4/1, checkMeasurementFcn4Signals/4
  Correct3/1 -> Correct4/4
  Correct4/1 -> [AfterCorrect]

== system main_RI_LIEKF_GNSSOutrage/State estimation/RI EKF_AOA_LSTM/Error State Kalman Filter/Simulink Function - GPS Measurements ==
  Rbn : Inport
  vn : Inport  Port=2
  pn : Inport  Port=3
  GPSMeasurementFcn_RIEKF : TriggerPort  TriggerType=function-call  IsSimulinkFunction=on  FunctionName=GPSMeasurementFcn_RIEKF  VariantControl=Variant
  Add : Sum
  Data Type Conversion1 : DataTypeConversion  OutDataTypeStr=single  SaturateOnIntegerOverflow=off  RndMeth=Floor
  MATLAB Function : MATLAB Function  TreatAsAtomicUnit=on
  MATLAB Function1 : MATLAB Function  Commented=on  TreatAsAtomicUnit=on
  Product : Product  Multiplication=Matrix(*)
  pn1 : InportShadow  Port=3
  vn1 : InportShadow  Port=2
  x : ArgIn  DisableCoverage=on  OutDataTypeStr=single  PortDimensions=state_dim  ArgumentName=x
  v : ArgIn  DisableCoverage=on  Port=2  OutDataTypeStr=single  PortDimensions=6  ArgumentName=v
  y : ArgOut  DisableCoverage=on  OutDataTypeStr=single  PortDimensions=6  ArgumentName=y
  wires:
  MATLAB Function/1(H) -> Data Type Conversion1/1
  Product/1 -> Add/1
  Add/1 -> y/1
  vn/1 -> MATLAB Function/1(vn)
  Rbn/1 -> MATLAB Function1/1(Rbn)
  vn1/1 -> MATLAB Function1/2(vn)
  pn1/1 -> MATLAB Function1/3(pn)
  x/1 -> Product/2
  v/1 -> Add/2
  pn/1 -> MATLAB Function/2(pn)
  Data Type Conversion1/1 -> Product/1

== system main_RI_LIEKF_GNSSOutrage/State estimation/RI EKF_AOA_LSTM/Error State Kalman Filter/Simulink Function - GPS Measurements1 ==
  vn : Inport
  pn : Inport  Port=2
  BaroMeasurementFcn_RIEKF : TriggerPort  TriggerType=function-call  IsSimulinkFunction=on  FunctionName=BaroMeasurementFcn_RIEKF  VariantControl=Variant
  Add : Sum
  Data Type Conversion1 : DataTypeConversion  OutDataTypeStr=single  SaturateOnIntegerOverflow=off  RndMeth=Floor
  MATLAB Function : MATLAB Function  TreatAsAtomicUnit=on
  Product : Product  Multiplication=Matrix(*)
  x : ArgIn  DisableCoverage=on  OutDataTypeStr=single  PortDimensions=state_dim  ArgumentName=x
  v : ArgIn  DisableCoverage=on  Port=2  OutDataTypeStr=single  PortDimensions=2  ArgumentName=v
  y : ArgOut  DisableCoverage=on  OutDataTypeStr=single  PortDimensions=2  ArgumentName=y
  wires:
  MATLAB Function/1(H_baro) -> Data Type Conversion1/1
  Product/1 -> Add/1
  Add/1 -> y/1
  vn/1 -> MATLAB Function/1(vn)
  x/1 -> Product/2
  v/1 -> Add/2
  pn/1 -> MATLAB Function/2(pn)
  Data Type Conversion1/1 -> Product/1

== system main_RI_LIEKF_GNSSOutrage/State estimation/RI EKF_AOA_LSTM/Error State Kalman Filter/Simulink Function - GPS Measurements2 ==
  Rbn : Inport
  Magn : Inport  Port=2
  xstate : Inport  Port=3
  MagnMeasurementFcn_RIEKF : TriggerPort  TriggerType=function-call  IsSimulinkFunction=on  FunctionName=MagnMeasurementFcn_RIEKF  VariantControl=Variant
  Add : Sum
  Data Type Conversion1 : DataTypeConversion  OutDataTypeStr=single  SaturateOnIntegerOverflow=off  RndMeth=Floor
  MATLAB Function : MATLAB Function  TreatAsAtomicUnit=on
  Product : Product  Multiplication=Matrix(*)
  Selector : Selector  InputPortWidth=state_dim  IndexOptions=Index vector (dialog)  Indices=[1 2 3]  OutputSizes=1
  x : ArgIn  DisableCoverage=on  OutDataTypeStr=single  PortDimensions=state_dim  ArgumentName=x
  v : ArgIn  DisableCoverage=on  Port=2  OutDataTypeStr=single  PortDimensions=3  ArgumentName=v
  y : ArgOut  DisableCoverage=on  OutDataTypeStr=single  PortDimensions=3  ArgumentName=y
  wires:
  MATLAB Function/1(H) -> Data Type Conversion1/1
  Product/1 -> Add/1
  Add/1 -> y/1
  Magn/1 -> MATLAB Function/2(Magn)
  x/1 -> Product/2
  v/1 -> Add/2
  Data Type Conversion1/1 -> Product/1
  Rbn/1 -> MATLAB Function/1(Rbn)
  xstate/1 -> Selector/1
  Selector/1 -> MATLAB Function/3(dtheta)

== system main_RI_LIEKF_GNSSOutrage/State estimation/RI EKF_AOA_LSTM/Error State Kalman Filter/Simulink Function - GPS Measurements3 ==
  Rbn : Inport
  vn : Inport  Port=2
  Rab : Inport  Port=3
  vel_wind_NED : Inport  Port=4
  AirspeedMeasurementFcn_RIEKF : TriggerPort  TriggerType=function-call  IsSimulinkFunction=on  FunctionName=AirspeedMeasurementFcn_RIEKF  VariantControl=Variant
  Add : Sum
  Data Type Conversion1 : DataTypeConversion  OutDataTypeStr=single  SaturateOnIntegerOverflow=off  RndMeth=Floor
  MATLAB Function : MATLAB Function  TreatAsAtomicUnit=on
  Product : Product  Multiplication=Matrix(*)
  x : ArgIn  DisableCoverage=on  OutDataTypeStr=single  PortDimensions=state_dim  ArgumentName=x
  v : ArgIn  DisableCoverage=on  Port=2  OutDataTypeStr=single  PortDimensions=3  ArgumentName=v
  y : ArgOut  DisableCoverage=on  OutDataTypeStr=single  PortDimensions=3  ArgumentName=y
  wires:
  MATLAB Function/1(H) -> Data Type Conversion1/1
  Product/1 -> Add/1
  Add/1 -> y/1
  x/1 -> Product/2
  v/1 -> Add/2
  Data Type Conversion1/1 -> Product/1
  Rbn/1 -> MATLAB Function/1(Rbn)
  vn/1 -> MATLAB Function/3(vn)
  Rab/1 -> MATLAB Function/2(Rab)
  vel_wind_NED/1 -> MATLAB Function/4(v_wind)

== system main_RI_LIEKF_GNSSOutrage/State estimation/RI EKF_AOA_LSTM/Error State Kalman Filter/Simulink Function - State Transition ==
  DCM_b_n : Inport
  vn : Inport  Port=2  PortDimensions=[3,1]
  pn : Inport  Port=3  PortDimensions=[3,1]
  stateTransitionFcn_RIEKF : TriggerPort  TriggerType=function-call  IsSimulinkFunction=on  FunctionName=stateTransitionFcn_RIEKF  VariantControl=Variant
  Add : Sum
  Cal Phi : Subsystem
  Constant : Constant  Value=dt  OutDataTypeStr=single
  Data Type Conversion1 : DataTypeConversion  OutDataTypeStr=single  SaturateOnIntegerOverflow=off  RndMeth=Floor
  Data Type Conversion6 : DataTypeConversion  OutDataTypeStr=single  SaturateOnIntegerOverflow=off  RndMeth=Floor
  MATLAB Function : MATLAB Function  TreatAsAtomicUnit=on
  Product1 : Product  Multiplication=Matrix(*)
  Product2 : Product  Multiplication=Matrix(*)
  x : ArgIn  DisableCoverage=on  OutDataTypeStr=single  PortDimensions=state_dim  ArgumentName=x
  w : ArgIn  Port=2  OutDataTypeStr=single  PortDimensions=cov_dim  ArgumentName=w
  xNext : ArgOut  DisableCoverage=on  OutDataTypeStr=single  PortDimensions=state_dim  ArgumentName=xNext
  wires:
  x/1 -> Product2/2
  Product2/1 -> Data Type Conversion6/1
  MATLAB Function/1(G) -> Product1/1
  w/1 -> Product1/2
  Product1/1 -> Data Type Conversion1/1
  Add/1 -> xNext/1
  [DCM_b_n] -> MATLAB Function/1(Rbn)
  Constant/1 -> MATLAB Function/4(dt)
  DCM_b_n/1 -> [DCM_b_n]
  Cal Phi/1(Phi) -> Product2/1
  Data Type Conversion6/1 -> Add/2
  [DCM_b_n] -> Cal Phi/1(Rbn)
  vn/1 -> MATLAB Function/2(vn), Cal Phi/2(vn)
  pn/1 -> MATLAB Function/3(pn), Cal Phi/3(pn)
  Data Type Conversion1/1 -> Add/1

== system main_RI_LIEKF_GNSSOutrage/State estimation/RI EKF_AOA_LSTM/Error State Kalman Filter/Simulink Function - State Transition1 ==
  DCM_b_n : Inport
  vn : Inport  Port=2  PortDimensions=[3,1]
  pn : Inport  Port=3  PortDimensions=[3,1]
  stateFcn_RIEKFJacobian : TriggerPort  TriggerType=function-call  IsSimulinkFunction=on  FunctionName=stateFcn_RIEKFJacobian  VariantControl=Variant
  Cal Phi : Subsystem
  Constant : Constant  Value=dt  OutDataTypeStr=single
  Data Type Conversion1 : DataTypeConversion  OutDataTypeStr=single  SaturateOnIntegerOverflow=off  RndMeth=Floor
  Data Type Conversion6 : DataTypeConversion  OutDataTypeStr=single  SaturateOnIntegerOverflow=off  RndMeth=Floor
  MATLAB Function : MATLAB Function  TreatAsAtomicUnit=on
  Terminator : Terminator
  Terminator1 : Terminator
  x : ArgIn  DisableCoverage=on  OutDataTypeStr=single  PortDimensions=state_dim  ArgumentName=x
  w : ArgIn  Port=2  OutDataTypeStr=single  PortDimensions=cov_dim  ArgumentName=w
  A : ArgOut  DisableCoverage=on  OutDataTypeStr=single  PortDimensions=[state_dim,state_dim]  ArgumentName=A
  G : ArgOut  Port=2  OutDataTypeStr=single  PortDimensions=[24,21]  ArgumentName=G
  wires:
  pn/1 -> Cal Phi/3(pn), MATLAB Function/3(pn)
  vn/1 -> Cal Phi/2(vn), MATLAB Function/2(vn)
  [DCM_b_n] -> Cal Phi/1(Rbn)
  DCM_b_n/1 -> [DCM_b_n]
  Constant/1 -> MATLAB Function/4(dt)
  [DCM_b_n] -> MATLAB Function/1(Rbn)
  w/1 -> Terminator/1
  x/1 -> Terminator1/1
  MATLAB Function/1(G) -> Data Type Conversion6/1
  Cal Phi/1(Phi) -> Data Type Conversion1/1
  Data Type Conversion6/1 -> G/1
  Data Type Conversion1/1 -> A/1
